simulink model "CLLC_2022"  (R2022b)
settings: Solver=ode4  StartTime=0.0  StopTime=0.2  FixedStep=1e-8  MaxStep=1e-6  RelTol=1e-3
undefined symbols (not defined in the file or in its folder): fn, magnitude, Rl
libraries: spsSeriesRLCBranchLib x9, spsMosfetLib x8, powerlib_extras x6, spsCurrentMeasurementLib x5, spsVoltageMeasurementLib x5, spsRMSLib x4, spsLinearTransformerLib x1, dspsigops x1, slpidlib x1, spsIdealSwitchLib x1, spsDCVoltageSourceLib x1, spspowerguiLib x1
settings Model: SimulationMode=accelerator  Creator=Administrator  LastModifiedBy=57792

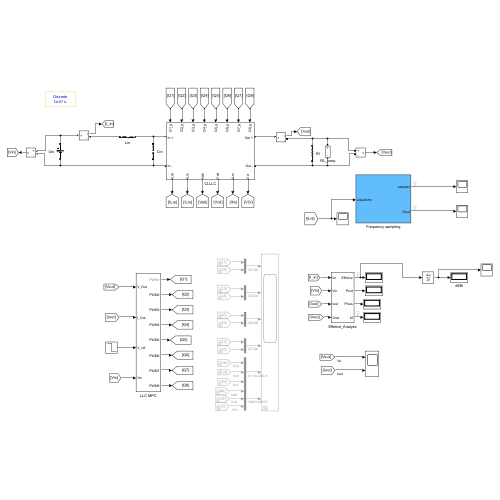
[thumbnail: Simulink's stored preview of the top-level diagram]
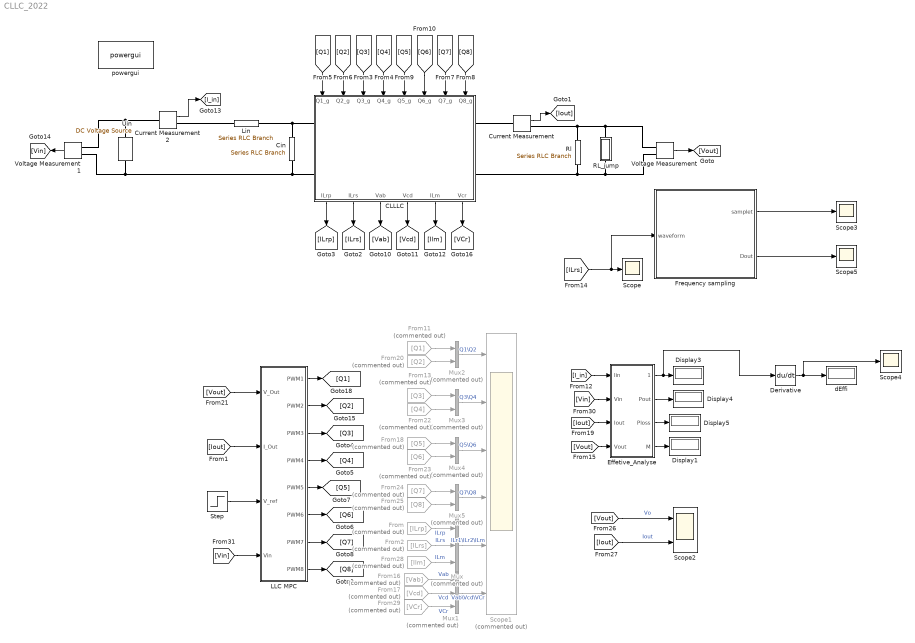
== system CLLC_2022 ==
  CLLLC : Subsystem
      settings: PortSchema="{\"entries\":[{\"content\":{\"sides\":[{\"content\":{\"connectorIds\":[\"LConn1\",\"LConn2\"]},\"type\":\"ConnectorPlacement.EquallySpacedRectSide\",\"uuid\":\"1ddeb927-71a3-4220-b338-aababa395dac\"},{\"content\":{\"connectorIds\":[\"RConn1\",\"RConn2\"],\"side\":\"RIGHT\"},\"type\":\"ConnectorPlacement.EquallySpacedRectSide\",\"uuid\":\"f8c4c052-3320-48db-aef8-ab942bc92f6b\"},{\"content\":{\"connectorIds\":[\"In1\",\"In2\",\"In3\",\"In4\",\"In5\",\"In6\",\"In7\",\"In8\"],\"side\":\"TOP\"},\"type\":\"ConnectorPlacement.EquallySpacedRectSide\",\"uuid\":\"8adaa841-f2db-435d-929f-b46912787eff\"},{\"content\":{\"connectorIds\":[\"Out1\",\"Out2\",\"Out3\",\"Out4\",\"Out5\",\"Out6\"],\"side\":\"BOTTOM\"},\"type\":\"ConnectorPlacement.EquallySpacedRectSide\",\"uuid\":\"70667971-f234-4810-a3f7-1e84327e61b9\"}]},\"type\":\"ConnectorPlacement.EquallySpacedConnector\",\"uuid\":\"6e5c2af6-c88b-4768-9377-4f05e38ffda3\"}],\"packageUris\":[\"http://schema.mathworks.com/mf0/Connector/R2020b\"],\"version\":\"1.0\"}"
  Cin : spsSeriesRLCBranchLib/Series RLC Branch  LConnTagsString=__new0  RConnTagsString=__new0  BranchType=C  Resistance=400  Inductance=10e-9  SetiL0=off  InitialCurrent=0  Capacitance=220e-6  Setx0=off  InitialVoltage=0  Measurements=None
  Current Measurement : spsCurrentMeasurementLib/Current Measurement  PhasorSimulation=off  OutputType=Complex  PSBequivalent=0
  Current Measurement2 : spsCurrentMeasurementLib/Current Measurement  PhasorSimulation=off  OutputType=Complex  PSBequivalent=0
  Derivative : Derivative
  Display{1,3..5} (4 alike) : Display
  Effetive_Analyse : Subsystem
  Frequency sampling : Subsystem
  From : From  Commented=on  GotoTag=ILrp
  From11 : From  Commented=on  GotoTag=Q1
  From13 : From  Commented=on  GotoTag=Q3
  From16 : From  Commented=on  GotoTag=Vab
  From17 : From  Commented=on  GotoTag=Vcd
  From18 : From  Commented=on  GotoTag=Q5
  From2 : From  Commented=on  GotoTag=ILrs
  From20 : From  Commented=on  GotoTag=Q2
  From22 : From  Commented=on  GotoTag=Q4
  From23 : From  Commented=on  GotoTag=Q6
  From24 : From  Commented=on  GotoTag=Q7
  From25 : From  Commented=on  GotoTag=Q8
  From28 : From  Commented=on  GotoTag=Ilm
  From29 : From  Commented=on  GotoTag=VCr
  LLC MPC : Subsystem  mask{Fn_Max=1, Fn_Min=1, Fs=160e3, Td=1e-7}
      mask prompts: Fn_Max "最大频率"; Fn_Min "最小频率"; Fs "谐振频率"; Td "死区时间"
      mask DialogControl ParameterGroupVar Prompt: 参数
  Lin : spsSeriesRLCBranchLib/Series RLC Branch  LConnTagsString=__new0  RConnTagsString=__new0  BranchType=RL  Resistance=0.01  Inductance=10e-9  SetiL0=off  InitialCurrent=0  Capacitance=2.2e-3  Setx0=off  InitialVoltage=0  Measurements=None
  Mux : Mux  Commented=on  Inputs=3
  Mux1 : Mux  Commented=on  Inputs=3
  Mux{2..5} (4 alike) : Mux  Commented=on  Inputs=2
  RL_jump : Subsystem  mask{RL=800, Tj=1}
      mask prompts: RL "R并联负载电阻"; Tj "Tj跳变时间"
      settings: PortSchema="{\"entries\":[{\"content\":{\"sides\":[{\"content\":{\"connectorIds\":[]},\"type\":\"ConnectorPlacement.EquallySpacedRectSide\",\"uuid\":\"4c795bd4-1bab-4c55-833f-6eced2a87930\"},{\"content\":{\"connectorIds\":[],\"side\":\"RIGHT\"},\"type\":\"ConnectorPlacement.EquallySpacedRectSide\",\"uuid\":\"14618bb5-b612-4b35-9ba9-216447f96e21\"},{\"content\":{\"connectorIds\":[\"LConn1\"],\"side\":\"TOP\"},\"type\":\"ConnectorPlacement.EquallySpacedRectSide\",\"uuid\":\"12a1c8ce-3ff4-42ff-a56b-3f4b2a897ee3\"},{\"content\":{\"connectorIds\":[\"RConn1\"],\"side\":\"BOTTOM\"},\"type\":\"ConnectorPlacement.EquallySpacedRectSide\",\"uuid\":\"f74f5f2e-d732-445c-972a-4bb2854aa00c\"}]},\"type\":\"ConnectorPlacement.EquallySpacedConnector\",\"uuid\":\"1c1d3e25-938c-4dd2-b079-0be3ce61fe3c\"}],\"packageUris\":[\"http://schema.mathworks.com/mf0/Connector/R2020b\"],\"version\":\"1.0\"}"
      mask DialogControl ParameterGroupVar Prompt: 参数
  Rl : spsSeriesRLCBranchLib/Series RLC Branch  LConnTagsString=__new0  RConnTagsString=__new0  BranchType=R  Resistance=Rl  Inductance=13e-6  SetiL0=off  InitialCurrent=0  Capacitance=2.2e-3  Setx0=off  InitialVoltage=0  Measurements=None
  Scope{,3..5} (4 alike) : Scope
  Scope1 : Scope  Commented=on  NumInputPorts=6
  Scope2 : Scope  NumInputPorts=2
  Step : Step  Before=460  After=400  SampleTime=0
  Uin : spsDCVoltageSourceLib/DC Voltage Source  Amplitude=400  Measurements=None
  Voltage Measurement : spsVoltageMeasurementLib/Voltage Measurement  PhasorSimulation=off  OutputType=Complex  PSBequivalent=0
  Voltage Measurement1 : spsVoltageMeasurementLib/Voltage Measurement  PhasorSimulation=off  OutputType=Complex  PSBequivalent=0
  dEffi : Display
  powergui : spspowerguiLib/powergui  Priority=1  SimulationMode=Discrete  SampleTime=1e-7  frequency=60  Iterations=50  frequencyindice=0  Pbase=100e6  ErrMax=1e-4  UnitsV=kV  UnitsW=MW  buscounter=0  FunctionMessages=off  echomessages=off  EnableUseOfTLC=off  CurrentSourceSwitches=off  DisableSnubberDevices=off  DisableRonSwitches=off  DisableVfSwitches=off  DisplayEquations=off  AutomaticDiscreteSolvers=off  SolverType=Tustin/Backward Euler (TBE)  Interpol=off  ExternalGateDelay=off  methode=off  Ts=100  x0status=blocks  SPID=on  SwTol=0  HookPort=off  NonlinearTolerance=1e-4  nMaxIteration=100  ContinueOnMaxIteration=off  RestoreLinks=warning  ResistiveCurrentMeasurement=off  Frange=[0:2:500]  Ylog=off  Xlog=on  ShowGrid=off  save=off  variable=ZData  structure=0  ZoomFFT=off  StartTime=0.0  cycles=1  DisplayStyle=1  fundamental=60  FreqAxis=off  MaxFrequency=1000  frequencyindicesteady=1  RmsSteady=1  display=off
  wires:
  Current Measurement/1 -> [Iout]
  Current Measurement2/1 -> [I_in]
  Voltage Measurement1/1 -> [Vin]
  [Q1] -> CLLLC/1(Q1_g)
  Voltage Measurement/1 -> [Vout]
  [Q2] -> CLLLC/2(Q2_g)
  [Vout] -> LLC MPC/1(V_Out)
  LLC MPC/2(PWM2) -> [Q2]
  LLC MPC/1(PWM1) -> [Q1]
  Step/1 -> LLC MPC/3(V_ref)
  [Iout] -> LLC MPC/2(I_Out)
  CLLLC/1(ILrp) -> [ILrp]
  CLLLC/2(ILrs) -> [ILrs]
  [Q3] -> CLLLC/3(Q3_g)
  [Q4] -> CLLLC/4(Q4_g)
  [Q5] -> CLLLC/5(Q5_g)
  [Q6] -> CLLLC/6(Q6_g)
  [Q7] -> CLLLC/7(Q7_g)
  [Q8] -> CLLLC/8(Q8_g)
  LLC MPC/3(PWM3) -> [Q3]
  LLC MPC/4(PWM4) -> [Q4]
  LLC MPC/5(PWM5) -> [Q5]
  LLC MPC/6(PWM6) -> [Q6]
  LLC MPC/7(PWM7) -> [Q7]
  LLC MPC/8(PWM8) -> [Q8]
  [Iout] -> Effetive_Analyse/3(Iout)
  [I_in] -> Effetive_Analyse/1(Iin)
  Effetive_Analyse/3(Ploss) -> Display5/1
  [Vin] -> Effetive_Analyse/2(Vin)
  [Vout] -> Effetive_Analyse/4(Vout)
  Effetive_Analyse/2(Pout) -> Display4/1
  Effetive_Analyse/1(Effetive) -> Derivative/1, Display3/1
  From2/1 -> Mux/2  "ILrs"
  From/1 -> Mux/1  "ILrp"
  From16/1 -> Mux1/1  "Vab"
  From17/1 -> Mux1/2  "Vcd"
  From11/1 -> Mux2/1
  From20/1 -> Mux2/2
  From13/1 -> Mux3/1
  From22/1 -> Mux3/2
  From18/1 -> Mux4/1
  From23/1 -> Mux4/2
  From24/1 -> Mux5/1
  From25/1 -> Mux5/2
  From28/1 -> Mux/3  "ILm"
  From29/1 -> Mux1/3  "VCr"
  Effetive_Analyse/4(M) -> Display1/1
  CLLLC/5(ILm) -> [Ilm]
  CLLLC/3(Vab) -> [Vab]
  CLLLC/4(Vcd) -> [Vcd]
  [Vout] -> Scope2/1  "Vo"
  CLLLC/6(Vcr) -> [VCr]
  [Iout] -> Scope2/2  "Iout"
  Mux2/1 -> Scope1/1  "Q1\\Q2"
  Mux3/1 -> Scope1/2  "Q3\\Q4"
  Mux4/1 -> Scope1/3  "Q5\\Q6"
  Mux5/1 -> Scope1/4  "Q7\\Q8"
  Mux/1 -> Scope1/5  "ILr1\\ILr2\\ILm"
  Mux1/1 -> Scope1/6  "Vab\\Vcd\\VCr"
  [Vin] -> LLC MPC/4(Vin)
  [ILrs] -> Frequency sampling/1(waveform), Scope/1
  Frequency sampling/1(samplet) -> Scope3/1
  Derivative/1 -> Scope4/1, dEffi/1
  Frequency sampling/2(Dout) -> Scope5/1
  connections:
  Rl/LConn1 -- Current Measurement/RConn1 -- RL_jump/LConn1 -- Voltage Measurement/LConn1
  Lin/LConn1 -- Cin/LConn1 -- CLLLC/LConn1
  CLLLC/RConn1 -- Current Measurement/LConn1
  CLLLC/LConn2 -- Voltage Measurement1/LConn2 -- Uin/LConn1 -- Cin/RConn1
  CLLLC/RConn2 -- Rl/RConn1 -- RL_jump/RConn1 -- Voltage Measurement/LConn2
  Voltage Measurement1/LConn1 -- Uin/RConn1 -- Current Measurement2/LConn1
  Current Measurement2/RConn1 -- Lin/RConn1

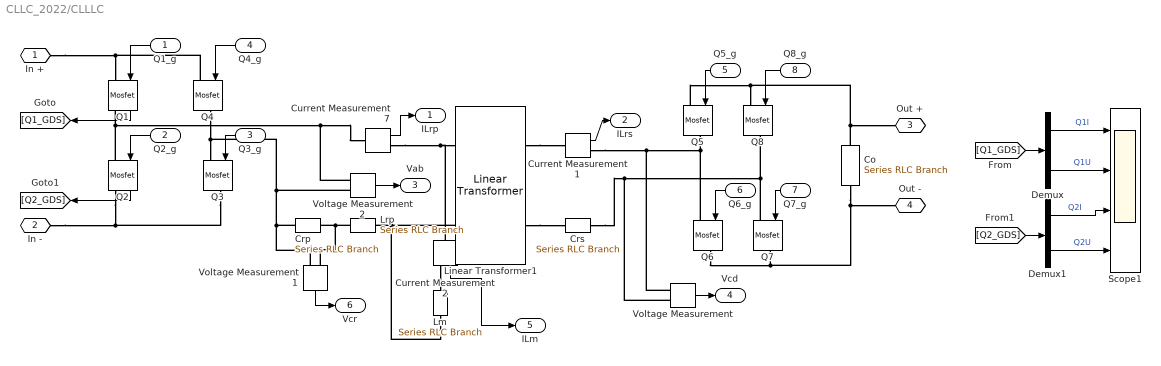
== system CLLC_2022/CLLLC ==
  Q1_g : Inport
  Q2_g : Inport  Port=2
  Q3_g : Inport  Port=3
  Q4_g : Inport  Port=4
  Q5_g : Inport  Port=5
  Q6_g : Inport  Port=6
  Q7_g : Inport  Port=7
  Q8_g : Inport  Port=8
  Co : spsSeriesRLCBranchLib/Series RLC Branch  LConnTagsString=__new0  RConnTagsString=__new0  BranchType=RC  Resistance=0.001  Inductance=13e-6  SetiL0=off  InitialCurrent=0  Capacitance=470e-6  Setx0=off  InitialVoltage=0  Measurements=None
  Crp : spsSeriesRLCBranchLib/Series RLC Branch  LConnTagsString=__new0  RConnTagsString=__new0  BranchType=C  Resistance=0.05  Inductance=30e-6  SetiL0=off  InitialCurrent=0  Capacitance=33e-9  Setx0=off  InitialVoltage=0  Measurements=None
  Crs : spsSeriesRLCBranchLib/Series RLC Branch  LConnTagsString=__new0  RConnTagsString=__new0  BranchType=RC  Resistance=0.05  Inductance=20e-6  SetiL0=off  InitialCurrent=0  Capacitance=33e-9  Setx0=off  InitialVoltage=0  Measurements=None
  Current Measurement1 : spsCurrentMeasurementLib/Current Measurement  PhasorSimulation=off  OutputType=Complex  PSBequivalent=0
  Current Measurement2 : spsCurrentMeasurementLib/Current Measurement  PhasorSimulation=off  OutputType=Complex  PSBequivalent=0
  Current Measurement7 : spsCurrentMeasurementLib/Current Measurement  PhasorSimulation=off  OutputType=Complex  PSBequivalent=0
  Demux : Demux  Outputs=2
  Demux1 : Demux  Outputs=2
  Linear Transformer1 : spsLinearTransformerLib/Linear Transformer  UNITS=SI  NominalPower=[100 50]  winding1=[1 0 0]  winding2=[1 0 30e-6]  ThreeWindings=off  winding3=[1 0 0]  RmLm=[1e12 inf]  Measurements=None  DataType=on
  Lm : spsSeriesRLCBranchLib/Series RLC Branch  LConnTagsString=__new0  RConnTagsString=__new0  BranchType=L  Resistance=0.05  Inductance=150e-6  SetiL0=off  InitialCurrent=0  Capacitance=33e-9  Setx0=off  InitialVoltage=0  Measurements=None
  Lrp : spsSeriesRLCBranchLib/Series RLC Branch  LConnTagsString=__new0  RConnTagsString=__new0  BranchType=RL  Resistance=0.05  Inductance=30e-6  SetiL0=off  InitialCurrent=0  Capacitance=33e-9  Setx0=off  InitialVoltage=0  Measurements=None
  Q1 : spsMosfetLib/Mosfet  Ron=0.27  Lon=0  Rd=1e-4  Vfd=1.8  IC=0  Rs=1e5  Cs=1e-10  Measurements=on
  Q2 : spsMosfetLib/Mosfet  Ron=0.27  Lon=0  Rd=1e-4  Vfd=1.8  IC=0  Rs=1e5  Cs=1e-10  Measurements=on
  Q3 : spsMosfetLib/Mosfet  Ron=0.27  Lon=0  Rd=1e-4  Vfd=1.8  IC=0  Rs=1e5  Cs=1e-10  Measurements=off
  Q4 : spsMosfetLib/Mosfet  Ron=0.27  Lon=0  Rd=1e-4  Vfd=1.8  IC=0  Rs=1e5  Cs=1e-10  Measurements=off
  Q{5..8} (4 alike) : spsMosfetLib/Mosfet  Ron=0.027  Lon=0  Rd=1e-4  Vfd=1.2  IC=0  Rs=1e5  Cs=1e-10  Measurements=off
  Scope1 : Scope  NumInputPorts=4
  Voltage Measurement : spsVoltageMeasurementLib/Voltage Measurement  PhasorSimulation=off  OutputType=Complex  PSBequivalent=0
  Voltage Measurement1 : spsVoltageMeasurementLib/Voltage Measurement  PhasorSimulation=off  OutputType=Complex  PSBequivalent=0
  Voltage Measurement2 : spsVoltageMeasurementLib/Voltage Measurement  PhasorSimulation=off  OutputType=Complex  PSBequivalent=0
  In + : PMIOPort  Side=Left
  In - : PMIOPort  Port=2  Side=Left
  Out + : PMIOPort  Port=3  Side=Right
  Out - : PMIOPort  Port=4  Side=Right
  ILrp : Outport
  ILrs : Outport  Port=2
  Vab : Outport  Port=3
  Vcd : Outport  Port=4
  ILm : Outport  Port=5
  Vcr : Outport  Port=6
  wires:
  Current Measurement7/1 -> ILrp/1
  Q1_g/1 -> Q1/1
  Q2_g/1 -> Q2/1
  Q3_g/1 -> Q3/1
  Q4_g/1 -> Q4/1
  Q5_g/1 -> Q5/1
  Q6_g/1 -> Q6/1
  Q7_g/1 -> Q7/1
  Q8_g/1 -> Q8/1
  Current Measurement1/1 -> ILrs/1
  Voltage Measurement/1 -> Vcd/1
  [Q1_GDS] -> Demux/1
  Demux/1 -> Scope1/1  "Q1I"
  Demux/2 -> Scope1/2  "Q1U"
  Demux1/1 -> Scope1/3  "Q2I"
  Demux1/2 -> Scope1/4  "Q2U"
  [Q2_GDS] -> Demux1/1
  Voltage Measurement2/1 -> Vab/1
  Current Measurement2/1 -> ILm/1
  Voltage Measurement1/1 -> Vcr/1
  Q1/1 -> [Q1_GDS]
  Q2/1 -> [Q2_GDS]
  connections:
  Q2/LConn1 -- Voltage Measurement2/LConn1 -- Current Measurement7/LConn1 -- Q1/RConn1
  Current Measurement7/RConn1 -- Current Measurement2/LConn1 -- Linear Transformer1/LConn1
  In +/RConn1 -- Q4/LConn1 -- Q1/LConn1
  Q6/LConn1 -- Voltage Measurement/LConn1 -- Current Measurement1/RConn1 -- Q5/RConn1
  Linear Transformer1/LConn2 -- Lm/RConn1 -- Lrp/RConn1
  In -/RConn1 -- Q3/RConn1 -- Q2/RConn1
  Q4/RConn1 -- Voltage Measurement2/LConn2 -- Voltage Measurement1/LConn2 -- Crp/LConn1 -- Q3/LConn1
  Co/LConn1 -- Q5/LConn1 -- Q8/LConn1 -- Out +/RConn1
  Linear Transformer1/RConn1 -- Current Measurement1/LConn1
  Q7/LConn1 -- Voltage Measurement/LConn2 -- Crs/RConn1 -- Q8/RConn1
  Co/RConn1 -- Q6/RConn1 -- Q7/RConn1 -- Out -/RConn1
  Linear Transformer1/RConn2 -- Crs/LConn1
  Current Measurement2/RConn1 -- Lm/LConn1
  Lrp/LConn1 -- Voltage Measurement1/LConn1 -- Crp/RConn1

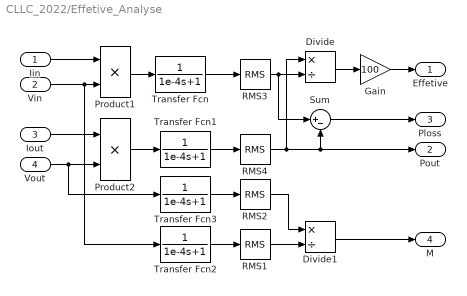
== system CLLC_2022/Effetive_Analyse ==
  Iin : Inport
  Vin : Inport  Port=2
  Iout : Inport  Port=3
  Vout : Inport  Port=4
  Divide : Product  Inputs=*/
  Divide1 : Product  Inputs=*/
  Gain : Gain  Gain=100
  Product1 : Product
  Product2 : Product
  RMS{1..4} (4 alike) : spsRMSLib/RMS  TrueRMS=on  Freq=1e3  RMSInit=0  Ts=0
  Sum : Sum  Inputs=|+-
  Transfer Fcn{,1..3} (4 alike) : TransferFcn  Denominator=[1e-4 1]
  Effetive : Outport
  Pout : Outport  Port=2
  Ploss : Outport  Port=3
  M : Outport  Port=4
  wires:
  RMS4/1 -> Divide/1, Sum/2, Pout/1
  Iin/1 -> Product1/1
  Divide/1 -> Gain/1
  Product2/1 -> Transfer Fcn1/1
  Product1/1 -> Transfer Fcn/1
  Vout/1 -> Transfer Fcn3/1, Product2/2
  Iout/1 -> Product2/1
  RMS3/1 -> Divide/2, Sum/1
  Transfer Fcn/1 -> RMS3/1
  Transfer Fcn1/1 -> RMS4/1
  Gain/1 -> Effetive/1
  Sum/1 -> Ploss/1
  Vin/1 -> Transfer Fcn2/1, Product1/2
  Transfer Fcn2/1 -> RMS1/1
  Transfer Fcn3/1 -> RMS2/1
  Divide1/1 -> M/1
  RMS2/1 -> Divide1/1
  RMS1/1 -> Divide1/2

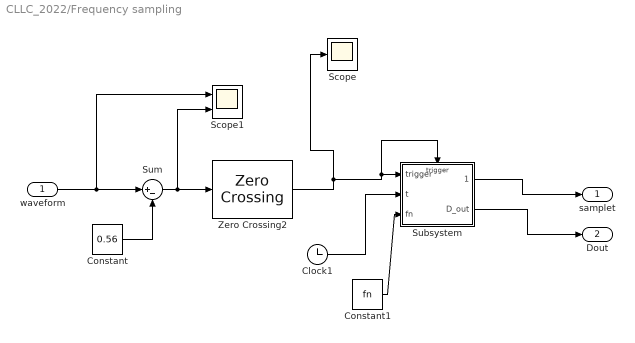
== system CLLC_2022/Frequency sampling ==
  waveform : Inport
  Clock1 : Clock
  Constant : Constant  Value=0.56
  Constant1 : Constant  Value=fn
  Scope : Scope
  Scope1 : Scope  NumInputPorts=2
  Subsystem : Subsystem
  Sum : Sum  Inputs=|+-
  Zero Crossing2 : dspsigops/Zero Crossing
  samplet : Outport
  Dout : Outport  Port=2
  wires:
  Zero Crossing2/1 -> Subsystem/Trigger, Subsystem/1(trigger), Scope/1
  Subsystem/1(delta_t_out) -> samplet/1
  Clock1/1 -> Subsystem/2(t)
  waveform/1 -> Scope1/1, Sum/1
  Sum/1 -> Scope1/2, Zero Crossing2/1
  Constant/1 -> Sum/2
  Subsystem/2(D_out) -> Dout/1
  Constant1/1 -> Subsystem/3(fn)

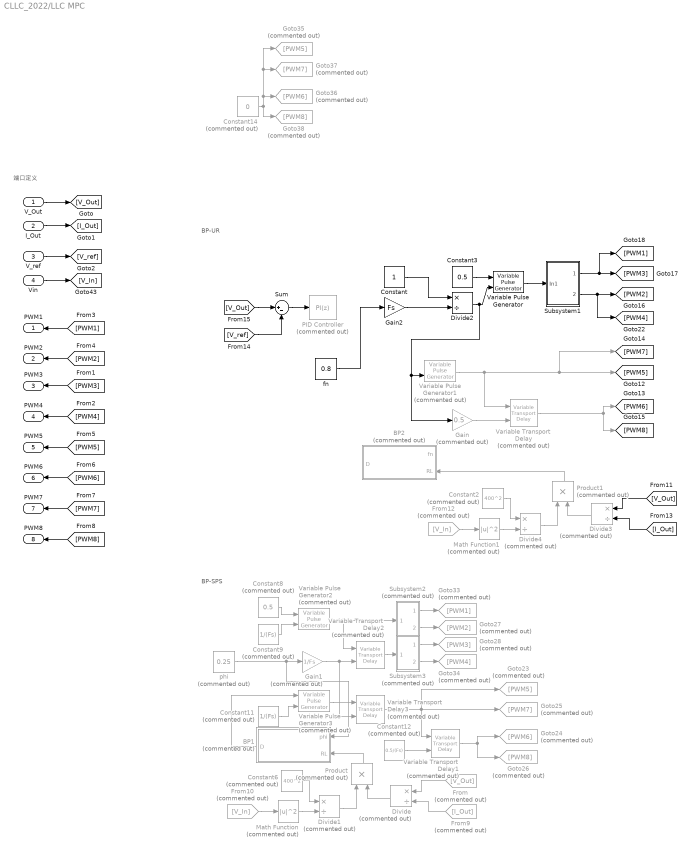
== system CLLC_2022/LLC MPC ==
  note: 端口定义
  note: BP-UR
  note: BP-SPS
  V_Out : Inport  SampleTime=1e-4
  I_Out : Inport  Port=2  SampleTime=1e-4
  V_ref : Inport  Port=3  SampleTime=1e-4
  Vin : Inport  Port=4  SampleTime=1e-4
  BP1 : MATLAB Function  Commented=on  TreatAsAtomicUnit=on
  BP2 : MATLAB Function  Commented=on  TreatAsAtomicUnit=on
  Constant : Constant
  Constant11 : Constant  Commented=on  Value=1/(Fs)
  Constant12 : Constant  Commented=on  Value=0.5/(Fs)
  Constant14 : Constant  Commented=on  Value=0
  Constant2 : Constant  Commented=on  Value=400^2
  Constant3 : Constant  Value=0.5
  Constant6 : Constant  Commented=on  Value=400^2
  Constant8 : Constant  Commented=on  Value=0.5
  Constant9 : Constant  Commented=on  Value=1/(Fs)
  Divide{,1,3..4} (4 alike) : Product  Commented=on  Inputs=*/
  Divide2 : Product  Inputs=*/
  From : From  Commented=on  GotoTag=V_Out
  From10 : From  Commented=on  GotoTag=V_In
  From12 : From  Commented=on  GotoTag=V_In
  From9 : From  Commented=on  GotoTag=I_Out
  Gain : Gain  Commented=on  Gain=0.5
  Gain1 : Gain  Commented=on  Gain=1/Fs
  Gain2 : Gain  Gain=Fs
  Goto23 : Goto  Commented=on  GotoTag=PWM5
  Goto24 : Goto  Commented=on  GotoTag=PWM6
  Goto25 : Goto  Commented=on  GotoTag=PWM7
  Goto26 : Goto  Commented=on  GotoTag=PWM8
  Goto27 : Goto  Commented=on  GotoTag=PWM2
  Goto28 : Goto  Commented=on  GotoTag=PWM3
  Goto33 : Goto  Commented=on  GotoTag=PWM1
  Goto34 : Goto  Commented=on  GotoTag=PWM4
  Goto35 : Goto  Commented=on  GotoTag=PWM5
  Goto36 : Goto  Commented=on  GotoTag=PWM6
  Goto37 : Goto  Commented=on  GotoTag=PWM7
  Goto38 : Goto  Commented=on  GotoTag=PWM8
  Math Function : Math  Commented=on  Operator=magnitude^2
  Math Function1 : Math  Commented=on  Operator=magnitude^2
  PID Controller : slpidlib/PID Controller  Commented=on  Controller=PI  Form=Parallel  TimeDomain=Discrete-time  UseExternalTs=off  SampleTime=1e-4  IntegratorMethod=Forward Euler  FilterMethod=Forward Euler  ControllerParametersSource=internal  P=1e-2  I=1e-1  UseKiTs=off  D=0  N=100  UseFilter=on  TunerSelectOption=Transfer Function Based (PID Tuner App)  InitialConditionSource=internal  InitialConditionForIntegrator=0.6  InitialConditionForFilter=0  DifferentiatorICPrevScaledInput=0  ExternalReset=none  TrackingMode=off  Kt=1  LimitOutput=on  SatLimitsSource=internal  UpperSaturationLimit=1  LowerSaturationLimit=0.6  LinearizeAsGain=on  AntiWindupMode=none  Kb=1  LimitIntegrator=on  UpperIntegratorSaturationLimit=1  LowerIntegratorSaturationLimit=0.6  POutMin=[]  POutMax=[]  IOutMin=[]  IOutMax=[]  DOutMin=[]  DOutMax=[]  NOutMin=[]  NOutMax=[]  SumOutMin=[]  SumOutMax=[]  SaturationOutMin=[]  SaturationOutMax=[]  PParamMin=[]  PParamMax=[]  IParamMin=[]  IParamMax=[]  DParamMin=[]  DParamMax=[]  NParamMin=[]  NParamMax=[]  KbParamMin=[]  KbParamMax=[]  KtParamMin=[]  KtParamMax=[]  KbOutMin=[]  KbOutMax=[]  KtOutMin=[]  KtOutMax=[]  IntegratorOutMin=[]  IntegratorOutMax=[]  FilterOutMin=[]  FilterOutMax=[]  SumI1OutMin=[]  SumI1OutMax=[]  SumI2OutMin=[]  SumI2OutMax=[]  SumI3OutMin=[]  SumI3OutMax=[]  SumI4OutMin=[]  SumI4OutMax=[]  SumDOutMin=[]  SumDOutMax=[]  DifferentiatorOutMin=[]  DifferentiatorOutMax=[]  FilterDiffOutCoefMin=[]  FilterDiffOutCoefMax=[]  ReciprocalOutMin=[]  ReciprocalOutMax=[]  SumDenOutMin=[]  SumDenOutMax=[]  SumNumOutMin=[]  SumNumOutMax=[]  DivideOutMin=[]  DivideOutMax=[]  UdiffTsProdOutMin=[]  UdiffTsProdOutMax=[]  NTsProdOutMin=[]  NTsProdOutMax=[]  UintegralTsProdOutMin=[]  UintegralTsProdOutMax=[]  UngainTsProdOutMin=[]  UngainTsProdOutMax=[]  IntegratorContinuousStateAttributes=''  IntegratorStateMustResolveToSignalObject=off  IntegratorRTWStateStorageClass=Auto  FilterContinuousStateAttributes=''  FilterStateMustResolveToSignalObject=off  FilterRTWStateStorageClass=Auto  ParallelPVariant=InternalParameters  IdealPVariant=Disabled  IVariant=InternalParameters  DVariant=Disabled  IntegratorVariant=Discrete  SatVariant=Enabled  AWVariant=Passthrough  PCopyVariant=Disabled  TRVariant=Disabled  FdbkBlocksVariant=Forward  IdealPFdbkVariant=Disabled  SatFdbkVariant=Disabled  DerivativeFilterVariant=Disabled  NVariant=Disabled  NCopyVariant=Disabled_SignalSpec  FilterICVariant=Disabled  IntegratorICVariant=InternalICs  ExternalResetVariant=Disabled  TRSumVariant=Passthrough  SumFdbkVariant=Disabled  SumVariant=Sum_PI  TsampFilterVariant=InternalTs  TsampNgainVariant=Passthrough  TsampIntegralVariant=Disabled_SignalSpec  ExternalSaturationOutDataTypeStr=Inherit: Same as second input
  Product : Product  Commented=on
  Product1 : Product  Commented=on
  Subsystem1 : Subsystem
  Subsystem2 : Subsystem  Commented=on
  Subsystem3 : Subsystem  Commented=on
  Sum : Sum  Inputs=|+-
  Variable Transport Delay{,1..3} (4 alike) : VariableTransportDelay  Commented=on  VariableDelayType=Variable transport delay  MaximumDelay=1000
  Variable Pulse Generator : VariablePulseGenerator  RunAtFixedTimeIntervals=on  SampleTime=1e-7
  Variable Pulse Generator1 : VariablePulseGenerator  Commented=on  SampleTime=0.1
  Variable Pulse Generator2 : VariablePulseGenerator  Commented=on  SampleTime=0.1
  Variable Pulse Generator3 : VariablePulseGenerator  Commented=on  SampleTime=0.1
  fn : Constant  Value=0.8
  phi : Constant  Commented=on  Value=0.25
  PWM1 : Outport
  PWM2 : Outport  Port=2
  PWM3 : Outport  Port=3
  PWM4 : Outport  Port=4
  PWM5 : Outport  Port=5
  PWM6 : Outport  Port=6
  PWM7 : Outport  Port=7
  PWM8 : Outport  Port=8
  wires:
  V_Out/1 -> [V_Out]
  I_Out/1 -> [I_Out]
  V_ref/1 -> [V_ref]
  [PWM1] -> PWM1/1
  [PWM2] -> PWM2/1
  [PWM4] -> PWM4/1
  [PWM3] -> PWM3/1
  [PWM6] -> PWM6/1
  [PWM5] -> PWM5/1
  [PWM8] -> PWM8/1
  [PWM7] -> PWM7/1
  Subsystem1/2(Out2) -> [PWM2], [PWM4]
  Variable Transport Delay/1 -> [PWM6], [PWM8]
  Subsystem1/1(Out1) -> [PWM1], [PWM3]
  Variable Pulse Generator/1 -> Subsystem1/1(In1)
  Constant3/1 -> Variable Pulse Generator/1
  Gain2/1 -> Divide2/2
  Variable Pulse Generator1/1 -> [PWM7], [PWM5], Variable Transport Delay/1
  Gain/1 -> Variable Transport Delay/2
  Constant12/1 -> Variable Transport Delay1/2
  BP1/1(D) -> Variable Pulse Generator3/1
  Constant9/1 -> Variable Pulse Generator2/2
  Variable Transport Delay1/1 -> Goto24/1, Goto26/1
  Constant11/1 -> Variable Pulse Generator3/2
  Constant8/1 -> Variable Pulse Generator2/1
  Variable Pulse Generator3/1 -> Variable Transport Delay3/1
  Variable Transport Delay3/1 -> Variable Transport Delay1/1, Goto25/1, Goto23/1
  Variable Pulse Generator2/1 -> Variable Transport Delay2/1, Subsystem2/1(In1)
  Subsystem2/1(Out1) -> Goto33/1
  Subsystem2/2(Out2) -> Goto27/1
  Variable Transport Delay2/1 -> Subsystem3/1(In1)
  Subsystem3/1(Out1) -> Goto28/1
  Subsystem3/2(Out2) -> Goto34/1
  Gain1/1 -> Variable Transport Delay3/2, Variable Transport Delay2/2
  Constant14/1 -> Goto38/1, Goto36/1, Goto37/1, Goto35/1
  phi/1 -> BP1/1(phi), Gain1/1
  From/1 -> Divide/1
  From9/1 -> Divide/2
  Vin/1 -> [V_In]
  From10/1 -> Math Function/1
  Math Function/1 -> Divide1/2
  Divide/1 -> Product/2
  Divide1/1 -> Product/1
  Product/1 -> BP1/2(RL)
  Constant6/1 -> Divide1/1
  Constant/1 -> Divide2/1
  Divide2/1 -> Gain/1, Variable Pulse Generator1/2, Variable Pulse Generator/2
  From12/1 -> Math Function1/1
  Math Function1/1 -> Divide4/2
  Constant2/1 -> Divide4/1
  [V_Out] -> Divide3/1
  [I_Out] -> Divide3/2
  Divide4/1 -> Product1/1
  Divide3/1 -> Product1/2
  Product1/1 -> BP2/2(RL)
  [V_Out] -> Sum/1
  [V_ref] -> Sum/2
  Sum/1 -> PID Controller/1
  fn/1 -> Gain2/1

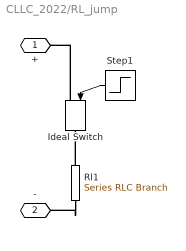
== system CLLC_2022/RL_jump ==
  Ideal Switch : spsIdealSwitchLib/Ideal Switch  Ron=0.001  Lon=0  IC=0  Rs=1e8  Cs=inf  Measurements=off
  Rl1 : spsSeriesRLCBranchLib/Series RLC Branch  LConnTagsString=__new0  RConnTagsString=__new0  BranchType=R  Resistance=RL  Inductance=13e-6  SetiL0=off  InitialCurrent=0  Capacitance=2.2e-3  Setx0=off  InitialVoltage=0  Measurements=None
  Step1 : Step  Time=Tj  SampleTime=0
  + : PMIOPort  Side=Left
  - : PMIOPort  Port=2  Side=Right
  wires:
  Step1/1 -> Ideal Switch/1
  connections:
  Ideal Switch/LConn1 -- +/RConn1
  Rl1/RConn1 -- -/RConn1
  Rl1/LConn1 -- Ideal Switch/RConn1

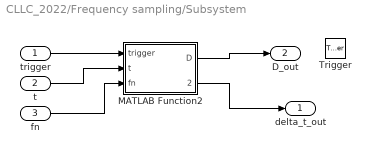
== system CLLC_2022/Frequency sampling/Subsystem ==
  trigger : Inport
  t : Inport  Port=2
  fn : Inport  Port=3
  Trigger : TriggerPort  VariantControl=(inherit)  PortDimensions=1
  MATLAB Function2 : MATLAB Function  TreatAsAtomicUnit=on
  delta_t_out : Outport
  D_out : Outport  Port=2
  wires:
  trigger/1 -> MATLAB Function2/1(trigger)
  MATLAB Function2/2(delta_t_out) -> delta_t_out/1
  t/1 -> MATLAB Function2/2(t)
  MATLAB Function2/1(D) -> D_out/1
  fn/1 -> MATLAB Function2/3(fn)

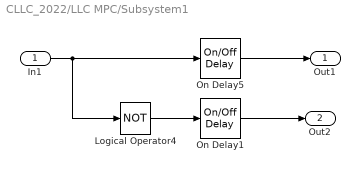
== system CLLC_2022/LLC MPC/Subsystem1 ==
  In1 : Inport
  Logical Operator4 : Logic  Operator=NOT  AllPortsSameDT=off  OutDataTypeStr=boolean
  On Delay1 : powerlib_extras/Control  Blocks/On//Off Delay  type_delay=On delay  delay=Td  ic=0
  On Delay5 : powerlib_extras/Control  Blocks/On//Off Delay  type_delay=On delay  delay=Td  ic=0
  Out1 : Outport
  Out2 : Outport  Port=2
  wires:
  On Delay5/1 -> Out1/1
  In1/1 -> On Delay5/1, Logical Operator4/1
  Logical Operator4/1 -> On Delay1/1
  On Delay1/1 -> Out2/1

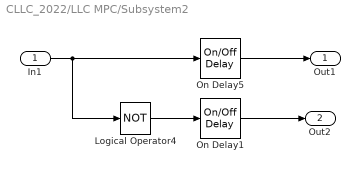
== system CLLC_2022/LLC MPC/Subsystem2 ==
  In1 : Inport
  Logical Operator4 : Logic  Operator=NOT  AllPortsSameDT=off  OutDataTypeStr=boolean
  On Delay1 : powerlib_extras/Control  Blocks/On//Off Delay  type_delay=On delay  delay=Td  ic=0
  On Delay5 : powerlib_extras/Control  Blocks/On//Off Delay  type_delay=On delay  delay=Td  ic=0
  Out1 : Outport
  Out2 : Outport  Port=2
  wires:
  On Delay5/1 -> Out1/1
  In1/1 -> On Delay5/1, Logical Operator4/1
  Logical Operator4/1 -> On Delay1/1
  On Delay1/1 -> Out2/1

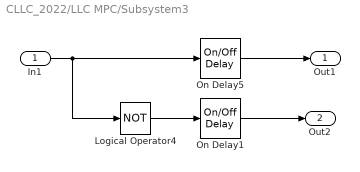
== system CLLC_2022/LLC MPC/Subsystem3 ==
  In1 : Inport
  Logical Operator4 : Logic  Operator=NOT  AllPortsSameDT=off  OutDataTypeStr=boolean
  On Delay1 : powerlib_extras/Control  Blocks/On//Off Delay  type_delay=On delay  delay=Td  ic=0
  On Delay5 : powerlib_extras/Control  Blocks/On//Off Delay  type_delay=On delay  delay=Td  ic=0
  Out1 : Outport
  Out2 : Outport  Port=2
  wires:
  On Delay5/1 -> Out1/1
  In1/1 -> On Delay5/1, Logical Operator4/1
  Logical Operator4/1 -> On Delay1/1
  On Delay1/1 -> Out2/1

== matlab function CLLC_2022/LLC MPC/BP2 ==
  data: fn input; D output; RL input
function D = UR_Network(fn,RL)

fn_n=5*fn-4;
RL_n=0.0022*RL-1.22;
x_in=[fn_n;RL_n];

W1=[-1.8033    0.0008
    0.9725    1.2256
    0.9993    0.0143];

W2=[0.1361    0.4091   -2.4660
   -0.3363    0.8031    0.6697];

b1=[1.0137
    2.0847
    1.3118];

b2=[1.1304
   -0.6780];

y=2./(1+exp(-2*(W1*x_in+b1)))-1;
y=W2*y+b2;

D=y(2,1)/9.5969+0.3956-0.1;

if(D>0.45) 
    D=0.45; 
elseif(D<0.05)
    D=0.05;
end

== matlab function CLLC_2022/Frequency sampling/Subsystem/MATLAB Function2 ==
  settings: updateMethod=DISCRETE
  data: D output; trigger input; delta_t_out output; t input; fn input
function [D,delta_t_out] = fcn(trigger,t,fn)
Ts = 1/(160e3*fn); %% 开关周期，其中fn在外部定义

persistent last_t;
persistent delta_t;
persistent last_delta_t;
if(isempty(last_t)||isempty(delta_t)||isempty(last_delta_t))
    last_t = 0;
    delta_t = 1;
    last_delta_t = 0;
end
if (trigger > 0 )
    delta_t = t - last_t;
    last_t = t;
    if (delta_t < Ts/2) %% 只有半个周期内的过零点才有效
      delta_t_out = delta_t;
      D = delta_t_out/Ts;
      last_delta_t = delta_t;
    else
      delta_t_out = last_delta_t;
      D = last_delta_t/Ts; 
    end
else
    delta_t_out = last_delta_t;
    D = last_delta_t/Ts; 
end

== matlab function CLLC_2022/LLC MPC/BP1 ==
  data: phi input; D output; RL input
function D = SPS_Network(phi,RL)

phi_n=5*phi-1;
RL_n=0.0022*RL-1.22;
x_in=[phi_n;RL_n];

W1=[0.3539   -0.0425
   -0.3619   -0.2712
   -0.4244    1.2797];

W2=[-36.3379   -2.1592   -0.6478
    9.8062    3.5222    0.8689];

b1=[-1.7429
    0.1982
   -0.3012];

b2=[-33.1925
    8.7709];

y=2./(1+exp(-2*(W1*x_in+b1)))-1;
y=W2*y+b2;

D=y(2,1)/6.2775+0.3394-0.1;


if(D>0.45) 
    D=0.45; 
elseif(D<0.05)
    D=0.05;
end
